simulink model "optsim1"  (Simulink 10.0)
settings: Solver=ode45  StartTime=0.0  StopTime=100  FixedStep=1  MaxStep=0.1  RelTol=1e-3  AbsTol=1e-6
PreLoadFcn:
  | a1=3; a2=43;
PostLoadFcn:
  | optsiminit
undefined symbols (not defined in the file): Kd, Kp
settings Model: Creator=nikita  LastModifiedBy=bhisma  ExtModeTrigMode=oneshot  ExtModeArmWhenConnect=off
settings SolverCC: AutoScaleAbsTol=off
settings DataIOCC: SignalLoggingSaveFormat=ModelDataLogs  SaveTime=off  StateSaveName=x  TimeSaveName=t
settings OptimizationCC: BooleanDataType=off  InitFltsAndDblsToZero=on
settings DebuggingCC: SaveWithParameterizedLinksMsg=none  SignalResolutionControl=TryResolveAllWithWarning  MultiTaskDSMMsg=warning  MultiTaskCondExecSysMsg=none  IntegerOverflowMsg=none  FcnCallInpInsideContextMsg=warning  IntegerSaturationMsg=none
settings HardwareCC: TargetUnknown=on
settings SFSimCC: SimUseLocalCustomCode=on  CustomCodeUndefinedFunction=FilterOut
settings RTWCC: RTWUseLocalCustomCode=on
settings GRTTargetCC: TargetFcnLib=ansi_tfl_tmw.mat

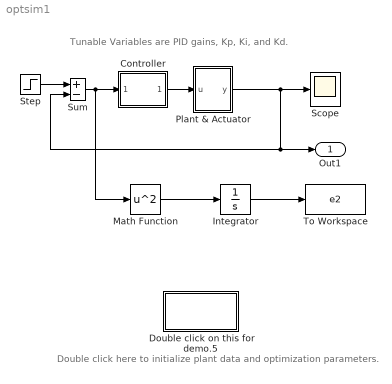
== system optsim1 ==
  note: Double click here to initialize plant data and optimization parameters.
  note: Tunable Variables are PID gains, Kp, Ki, and Kd.
  Controller : Subsystem  mask(PID Controller){P=Kp, I=0, D=Kd}
      mask prompts: P "Proportional:"; I "Integral"; D "Derivative:"
      mask help: Enter expressions for proportional, integral, and derivative terms.
      mask Help: This block implements a PID controller where paramaters are entered for the Proportional, Integral and Derivative terms.
      mask Display: disp('PID')
  Double click on this for demo.5 : Subsystem
      settings: OpenFcn=optsiminit
      mask Display: disp('optsiminit')
  Integrator : Integrator
  Math Function : Math  Operator=square  SaturateOnIntegerOverflow=on
  Plant & Actuator : Subsystem
  Scope : Scope
  Step : Step  Time=0  SampleTime=0
  Sum : Sum  Inputs=+-  SaturateOnIntegerOverflow=on  InputSameDT=on  OutDataTypeStr=Inherit: Same as first input
  To Workspace : ToWorkspace  VariableName=e2  SampleTime=-1
      settings: MaxDataPoints=1
  Out1 : Outport
  wires:
  Plant & Actuator/1(y) -> Sum/2, Out1/1, Scope/1
  Sum/1 -> Controller/1(In_1), Math Function/1
  Step/1 -> Sum/1
  Controller/1(Out_1) -> Plant & Actuator/1("u ")
  Math Function/1 -> Integrator/1
  Integrator/1 -> To Workspace/1

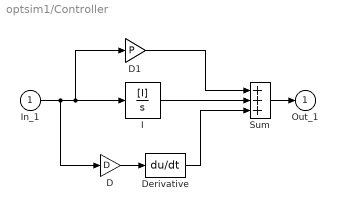
== system optsim1/Controller ==
  In_1 : Inport
  D : Gain  Gain=D  SaturateOnIntegerOverflow=on  OutDataTypeStr=Inherit: Same as input  ParamDataTypeStr=Inherit: Same as input
  D1 : Gain  Gain=P  SaturateOnIntegerOverflow=on  OutDataTypeStr=Inherit: Same as input  ParamDataTypeStr=Inherit: Same as input
  Derivative : Derivative
  I : TransferFcn  Numerator=[I]  Denominator=[1 0]
  Sum : Sum  Inputs=+++  SaturateOnIntegerOverflow=on  InputSameDT=on  OutDataTypeStr=Inherit: Same as first input
  Out_1 : Outport  InitialOutput=0
  wires:
  In_1/1 -> D1/1, I/1, D/1
  Sum/1 -> Out_1/1
  D/1 -> Derivative/1
  Derivative/1 -> Sum/3
  I/1 -> Sum/2
  D1/1 -> Sum/1

== system optsim1/Double click on this for demo.5 ==

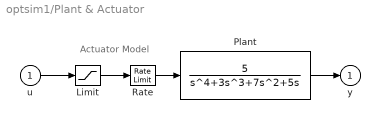
== system optsim1/Plant & Actuator ==
  note: Actuator Model
  "u " : Inport
  Limit : Saturate  UpperLimit=2  LowerLimit=-2
  Plant : TransferFcn  Numerator=[5]  Denominator=[1 3 7 5 0]
  Rate : RateLimiter  RisingSlewLimit=0.8  FallingSlewLimit=-0.8
  y : Outport  InitialOutput=0
  wires:
  Plant/1 -> y/1
  "u "/1 -> Limit/1
  Rate/1 -> Plant/1
  Limit/1 -> Rate/1
